simulink model "dc_motor_tf"  (R2018a)
settings: Solver=ode15s  StartTime=0.0  StopTime=50.0  RelTol=1e-3  EnableMultiTasking=on
PreLoadFcn:
  | J = 6;
  | L = 1e-6;
  | R = 0.3;
  | k = 0.5;
  | K = 0.5;
settings Model: Creator=jrivitus  LastModifiedBy=bneiswan
settings DataIOCC: SaveFormat=Array
settings OptimizationCC: ExpressionDepthLimit=2147483647  LifeSpan=inf
settings DebuggingCC: UnderspecifiedInitializationDetection=Classic  MergeDetectMultiDrivingBlocksExec=none  ParameterPrecisionLossMsg=none  FcnCallInpInsideContextMsg=warning  AllowSymbolicDim=off  StateNameClashWarn=warning  SFUnexpectedBacktrackingDiag=warning  SFNoUnconditionalDefaultTransitionDiag=warning  SFExecutionAtInitializationDiag=none
settings HardwareCC: ProdBitPerPointer=32  ProdBitPerSizeT=32  ProdBitPerPtrDiffT=32  ProdLargestAtomicFloat=None  ProdIntDivRoundTo=Undefined  ProdEndianess=Unspecified  ProdWordSize=32  ProdHWDeviceType=32-bit Generic
settings ModelReferenceCC: PropagateSignalLabelsOutOfModel=off
settings CodeAppCC: StateflowObjectComments=on
settings GRTTargetCC: TargetLangStandard=C89/C90 (ANSI)  GeneratePreprocessorConditionals=Disable all  CombineOutputUpdateFcns=off  GRTInterface=on
settings ConfigComp: CovMetricSettings=dw  CovHtmlReporting=on  CovSaveCumulativeToWorkspaceVar=on  CovSaveSingleToWorkspaceVar=on  CovExternalEMLEnable=off  CovSFcnEnable=off

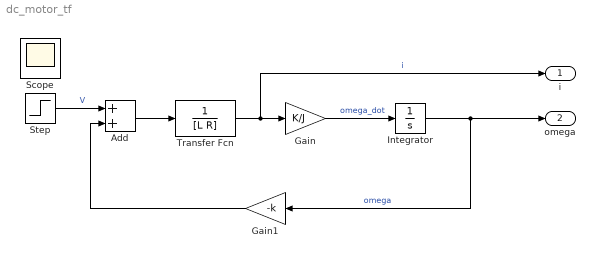
== system dc_motor_tf ==
  Add : Sum
  Gain : Gain  Gain=K/J
  Gain1 : Gain  Gain=-k
  Integrator : Integrator
  Step : Step  SampleTime=0
  Transfer Fcn : TransferFcn  Denominator=[L R]
  i : Outport
  omega : Outport  Port=2
  Scope : Scope
  wires:
  Integrator/1 -> Gain1/1, omega/1  "omega"
  Gain/1 -> Integrator/1  "omega_dot"
  Gain1/1 -> Add/2
  Step/1 -> Add/1  "V"
  Add/1 -> Transfer Fcn/1
  Transfer Fcn/1 -> Gain/1, i/1  "i"
